simulink model "WebCamTemp"  (Simulink 8.6)
settings: Solver=FixedStepDiscrete  StartTime=0.0  StopTime=Inf  RelTol=1e-3
values from neighbouring files (symbols this model uses):
  gain = 1.0    (= 1)    [WebCamTemp_param.m]
  H = 480    [WebCamTemp_param.m]
  Int = Int/max(max(Int))    [WebCamTemp_param.m]
  maxT = 25    [WebCamTemp_param.m]
  minT = 20    [WebCamTemp_param.m]
  mycmap = [0 0 0 0 0 0 0 0 0 0 0 0 ... (192 elements, 64x3)]    [MyColormaps.mat]
  nAvr = 8    [WebCamTemp_param.m]
  Op = Op/max(max(Op))    [WebCamTemp_param.m]
  T = 0.3    [WebCamTemp_param.m]
  W = 640    [WebCamTemp_param.m]
undefined symbols (not defined in the file or in its folder): IsPositionTracked, IsSkeletonTracked, JointDepthIndices, JointImageIndices, JointTrackingState, JointWorldCoordinates, none, PositionDepthIndices, PositionImageIndices, PositionWorldCoordinates, SegmentationData, serial, SkeletonTrackingID, videoinput
libraries: simulink x20, dspsigops x18, visionsinks x3, instrumentlib x3, visiontextngfix x2, dspstat3 x2, dspmtrx3 x2, visionstatistics x2, dspswit3 x1, powerlib_meascontrol x1, dspvision x1, imaqlib x1
settings Model: Creator=Valentina  LastModifiedBy=VIKTOR
settings OptimizationCC: DefaultParameterBehavior=Inlined
settings DebuggingCC: FcnCallInpInsideContextMsg=UseLocalSettings
settings HardwareCC: ProdBitPerPointer=64  ProdLargestAtomicFloat=Float  ProdIntDivRoundTo=Zero  ProdEndianess=LittleEndian  ProdWordSize=64  ProdHWDeviceType=Intel->x86-64 (Windows64)
settings GRTTargetCC: RTWCAPISignals=on  RTWCAPIParams=on
settings SimEventsCC: propDiagAttribOutput=1  propDiagFcnCallOutput=1  propDiagStatOutput=0  propPreventDuplicateEvents=0

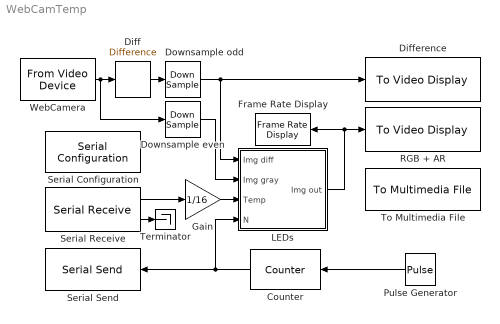
== system WebCamTemp ==
  Counter : dspswit3/Counter  Direction=Up  CountEvent=Rising edge  CounterSize=User defined  MaxCount=5  InitialCount=0  Output=Count  HitValue=32  ResetInput=off  SamplesPerFrame=1  Ts=1/30  CntDtype=uint8  HitDtype=Logical
  Diff : simulink/Discrete/Difference  ICPrevInput=0.0  InputProcessing=Inherited  OutMin=[]  OutMax=[]  OutDataType=fixdt(1, 16)  OutScaling=2^-10  DoSatur=off
  Difference : visionsinks/To Video Display  windowSizeMode=Normal  openAtMdlStart=on  fullScreen=off  videoWindowX=1204  videoWindowY=269  saveWindowSize=off  videoWindowWidth=640  videoWindowHeight=480  inputColorFormat=RGB  inputType=Obsolete  imagePorts=One multidimensional signal  OutputDevice=On-screen video monitor  dataOrg=Column-major  isWindowOpen=off
  "Downsample even " : DownSample
  Downsample odd : DownSample  phase=1
  Frame Rate Display : visionsinks/Frame Rate Display  UpdateRate=10
  Gain : Gain  Gain=1/16  OutDataTypeStr=double
  LEDs : Subsystem
  Pulse Generator : DiscretePulseGenerator  PhaseDelay=2  SampleTime=1/30
  RGB + AR : visionsinks/To Video Display  windowSizeMode=Normal  openAtMdlStart=on  fullScreen=off  videoWindowX=307  videoWindowY=272  saveWindowSize=off  videoWindowWidth=640  videoWindowHeight=480  inputColorFormat=RGB  inputType=Obsolete  imagePorts=One multidimensional signal  OutputDevice=On-screen video monitor  dataOrg=Column-major  isWindowOpen=off
  Serial Configuration : instrumentlib/Serial Configuration  Priority=-200000  ComPortMenu=COM9  ComPort=COM9  ObjConstructor=serial('COM9');  BaudRate=250000  DataBits=8  Parity=none  StopBits=1  FlowControl=none  Timeout=2  ByteOrder=LittleEndian
  Serial Receive : instrumentlib/Serial Receive  ComPortMenu=<Please select a port...>  ComPort=<Please select a port...>  Terminator=<none>  DataSize="[6  1]"  DataType=int16  EnableBlockingMode=off  ActionDataUnavailable=Output last received value  CustomValue=0  SampleTime=1/30
  Serial Send : instrumentlib/Serial Send  ComPortMenu=COM9  ComPort=COM9  ObjConstructor=serial('COM9');  Terminator=<none>  EnableBlockingMode=on
  Terminator : Terminator
  To Multimedia File : dspvision/To Multimedia File  outputFilename=F:\Matlab\WebCamTemp\output.mp4  streamSelection=Video only  videoCompressor=MJPEG Compressor  audioCompressor=None (uncompressed)  imagePorts=One multidimensional signal  fileType=MPEG4  audioDatatype=Determine from input data type  fourcc=RGB  videoQuality=100  mj2000CompFactor=10
  WebCamera : imaqlib/From Video Device  DeviceMenu=winvideo 1 (Webcam C170)  Device=winvideo 1 (Webcam C170)  ObjConstructor=videoinput('winvideo', 1)  VideoFormatMenu=YUY2_640x480  VideoFormat=YUY2_640x480  VideoSource=input1  ROIPosition=[0 0 480 640]  EnableHWTrigger=off  TriggerConfiguration=none/none  SampleTime=1/30  OutputPortsMode=One multidimensional signal  DataType=single  CanDoHWTrigger=no  ReturnedColorSpace=grayscale  BlockHandle=464.0011  ROIWidth=640  ROIHeight=480  ROIColumn=0  ROIRow=0  EngXMLPath=C:\Program Files\MATLAB\R2015b\toolbox\imaq\imaq\private  DevXMLPath=C:\MATLAB\SupportPackages\R2015b\osgenericvideointerface\toolbox\imaq\supportpackages\genericvideo\adaptor\win64  EngLibPath=C:\Program Files\MATLAB\R2015b\toolbox\imaq\imaqblks\imaqmex\win64  ColorSpace=grayscale  BayerSensorAlignment=grbg  AllMetadata=IsPositionTracked;IsSkeletonTracked;JointDepthIndices;JointImageIndices;JointTrackingState;JointWorldCoordinates;PositionDepthIndices;PositionImageIndices;PositionWorldCoordinates;SegmentationData;SkeletonTrackingID
  wires:
  Serial Receive/1 -> Gain/1
  Gain/1 -> LEDs/3(Temp)
  "Downsample even "/1 -> LEDs/2("Img gray ")
  Diff/1 -> Downsample odd/1
  Downsample odd/1 -> Difference/1, LEDs/1(Img diff)
  WebCamera/1 -> Diff/1, "Downsample even "/1
  Pulse Generator/1 -> Counter/1
  LEDs/1(Img out) -> Frame Rate Display/1, RGB + AR/1
  Serial Receive/2 -> Terminator/1
  Counter/1 -> LEDs/4(N), Serial Send/1

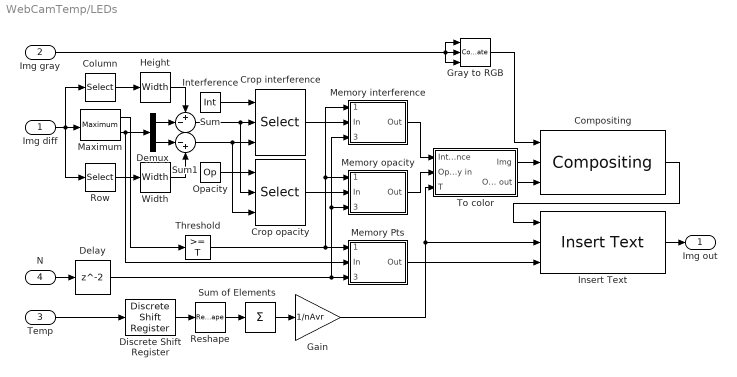
== system WebCamTemp/LEDs ==
  Img diff : Inport
  "Img gray " : Inport  Port=2
  Temp : Inport  Port=3
  N : Inport  Port=4
  Column : Selector  NumberOfDimensions=2  InputPortWidth=3  IndexOptions=Select all,Index vector (dialog)  Indices=1,1  OutputSizes=1,1
  Compositing : visiontextngfix/Compositing  operation=Blend  bFacSrc=Input port  mFacSrc=Specify via dialog  bFactor=0.75  mFactor=1  source=Specify via dialog  coordinates=[1 1]  prodOutputMode=Binary point scaling  prodOutputWordLength=32  prodOutputFracLength=10  roundingMode=Floor  overflowMode=off
  Crop interference : Selector  NumberOfDimensions=2  IndexMode=Zero-based  InputPortWidth=3  IndexOptions=Starting index (port),Starting index (port)  Indices=[1 3],1  OutputSizes=H,W
  Crop opacity : Selector  NumberOfDimensions=2  IndexMode=Zero-based  InputPortWidth=3  IndexOptions=Starting index (port),Starting index (port)  Indices=[1 3],1  OutputSizes=H,W
  Delay : Delay  InitialCondition=0
  Demux : Demux  Outputs=2
  Discrete Shift Register : powerlib_meascontrol/Additional Components/Discrete Shift Register  NSamples=nAvr  InitialValue=0  Ts=-1
  Gain : Gain  Gain=1/nAvr  OutDataTypeStr=single
  Gray to RGB : Concatenate  NumInputs=3  Mode=Multidimensional array  ConcatenateDimension=3
  Height : Width  DataType=uint32
  Insert Text : visiontextngfix/Insert Text  inputType=Obsolete  theText='%4.1f'  getTextLocFrom=Input port  textLoc=[1 1]  getTextColorFrom=Specify via dialog  textColor=[0 0 0]  getTextIntensityFrom=Specify via dialog  textIntensity=0  getTextOpacityFrom=Specify via dialog  textOpacity=1.0  dummyVar2=0  dummyVar3=0  dummyVar4=0  imagePorts=One multidimensional signal  isInputTransposed=off  fontFace=Arial  dummyVar1=0  blockFontSize=24  antiAliased=on
  Interference : Constant  Value=Int  OutDataTypeStr=single
  Maximum : dspstat3/Maximum  fcn=Value and Index  reset=None  indexBase=Zero  operateOver=Entire input  Dimension=1  operation=maximum  roiEnable=off  roiType=Rectangles  roiPortion=Entire ROI  roiOutput=Individual statistics for each ROI  roiFlag=off  accumDataTypeStr=Inherit: Same as product output  accumLastDataTypeStr=Inherit: Same as product output  roundingMode=Floor  overflowMode=off
  Memory interference : Subsystem
  Memory opacity : Subsystem
  Memory Pts : Subsystem
  Opacity : Constant  Value=Op  OutDataTypeStr=single
  Reshape : Reshape  OutputDimensionality=Customize  OutputDimensions=[nAvr,6]
  Row : Selector  NumberOfDimensions=2  InputPortWidth=3  IndexOptions=Index vector (dialog),Select all  Indices=1,1  OutputSizes=1,1
  Sum : Sum  Inputs=+-|
  Sum of Elements : Sum  Inputs=+  CollapseMode=Specified dimension
  Sum1 : Sum  Inputs=|-+
  Threshold : simulink/Logic and Bit Operations/Compare To Constant  relop=>=  const=T  OutDataTypeStr=boolean
  To color : Subsystem
  Width : Width  DataType=uint32
  Img out : Outport
  wires:
  Insert Text/1 -> Img out/1
  Compositing/1 -> Insert Text/1
  To color/2(Opacity out) -> Compositing/3
  Temp/1 -> Discrete Shift Register/1
  To color/1(Img) -> Compositing/2
  Interference/1 -> Crop interference/1
  Demux/2 -> Sum1/1
  Demux/1 -> Sum/2
  Height/1 -> Sum/1
  Sum/1 -> Crop opacity/2, Crop interference/2
  Sum1/1 -> Crop opacity/3, Crop interference/3
  Img diff/1 -> Maximum/1, Column/1, Row/1
  Memory interference/1(Out) -> To color/1(Interference)
  Memory opacity/1(Out) -> To color/2(Opacity in)
  Memory Pts/1(Out) -> Insert Text/3
  Row/1 -> Width/1
  Width/1 -> Sum1/2
  Column/1 -> Height/1
  N/1 -> Delay/1
  Maximum/2 -> Demux/1, Memory Pts/2(In)
  Maximum/1 -> Threshold/1
  Delay/1 -> Memory interference/3(Address), Memory opacity/3(Address), Memory Pts/3(Address)
  Opacity/1 -> Crop opacity/1
  Crop interference/1 -> Memory interference/2(In)
  Crop opacity/1 -> Memory opacity/2(In)
  Sum of Elements/1 -> Gain/1
  Discrete Shift Register/1 -> Reshape/1
  Reshape/1 -> Sum of Elements/1
  Gain/1 -> To color/3(T), Insert Text/2
  "Img gray "/1 -> Gray to RGB/3, Gray to RGB/1, Gray to RGB/2
  Gray to RGB/1 -> Compositing/1
  Threshold/1 -> Memory Pts/1(Enable), Memory interference/1(Enable), Memory opacity/1(Enable)

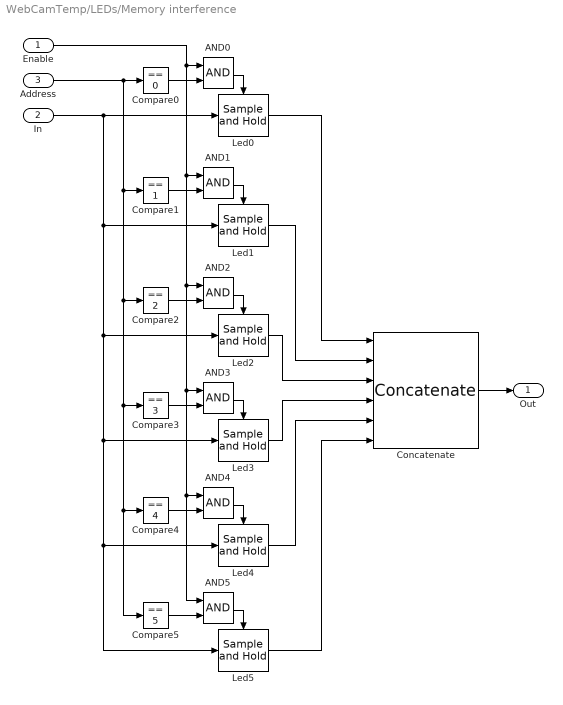
== system WebCamTemp/LEDs/Memory interference ==
  Enable : Inport
  In : Inport  Port=2
  Address : Inport  Port=3
  AND{0..5} (6 alike) : Logic  AllPortsSameDT=off  OutDataTypeStr=boolean
  Compare0 : simulink/Logic and Bit Operations/Compare To Constant  relop===  const=0  OutDataTypeStr=boolean
  Compare1 : simulink/Logic and Bit Operations/Compare To Constant  relop===  const=1  OutDataTypeStr=boolean
  Compare2 : simulink/Logic and Bit Operations/Compare To Constant  relop===  const=2  OutDataTypeStr=boolean
  Compare3 : simulink/Logic and Bit Operations/Compare To Constant  relop===  const=3  OutDataTypeStr=boolean
  Compare4 : simulink/Logic and Bit Operations/Compare To Constant  relop===  const=4  OutDataTypeStr=boolean
  Compare5 : simulink/Logic and Bit Operations/Compare To Constant  relop===  const=5  OutDataTypeStr=boolean
  Concatenate : Concatenate  NumInputs=6  Mode=Multidimensional array  ConcatenateDimension=3
  Led{0..5} (6 alike) : dspsigops/Sample and Hold  trig=Rising edge  initCond=0  latchinput=off
  Out : Outport
  wires:
  Address/1 -> Compare1/1, Compare2/1, Compare3/1, Compare4/1, Compare5/1, Compare0/1
  Concatenate/1 -> Out/1
  In/1 -> Led1/1, Led2/1, Led3/1, Led4/1, Led5/1, Led0/1
  AND0/1 -> Led0/Trigger
  Enable/1 -> AND5/1, AND4/1, AND3/1, AND2/1, AND1/1, AND0/1
  Compare0/1 -> AND0/2
  AND1/1 -> Led1/Trigger
  Compare1/1 -> AND1/2
  AND2/1 -> Led2/Trigger
  Compare2/1 -> AND2/2
  AND3/1 -> Led3/Trigger
  Compare3/1 -> AND3/2
  AND4/1 -> Led4/Trigger
  Compare4/1 -> AND4/2
  AND5/1 -> Led5/Trigger
  Compare5/1 -> AND5/2
  Led5/1 -> Concatenate/6
  Led0/1 -> Concatenate/1
  Led1/1 -> Concatenate/2
  Led4/1 -> Concatenate/5
  Led3/1 -> Concatenate/4
  Led2/1 -> Concatenate/3

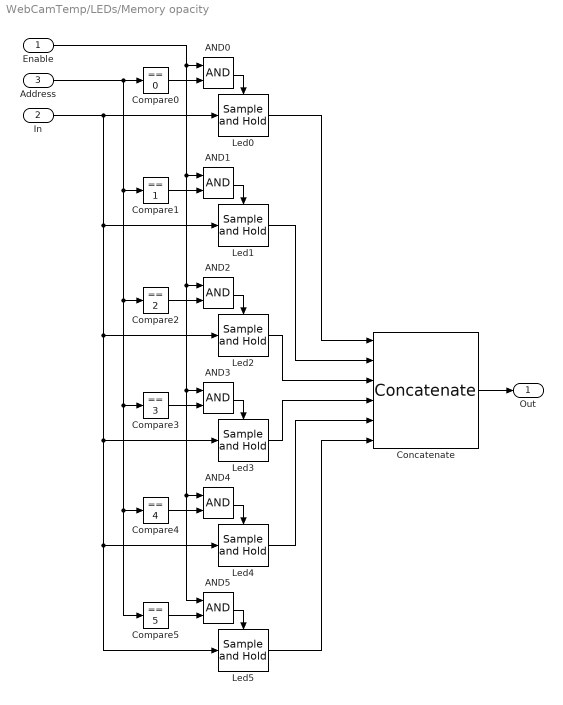
== system WebCamTemp/LEDs/Memory opacity ==
  Enable : Inport
  In : Inport  Port=2
  Address : Inport  Port=3
  AND{0..5} (6 alike) : Logic  AllPortsSameDT=off  OutDataTypeStr=boolean
  Compare0 : simulink/Logic and Bit Operations/Compare To Constant  relop===  const=0  OutDataTypeStr=boolean
  Compare1 : simulink/Logic and Bit Operations/Compare To Constant  relop===  const=1  OutDataTypeStr=boolean
  Compare2 : simulink/Logic and Bit Operations/Compare To Constant  relop===  const=2  OutDataTypeStr=boolean
  Compare3 : simulink/Logic and Bit Operations/Compare To Constant  relop===  const=3  OutDataTypeStr=boolean
  Compare4 : simulink/Logic and Bit Operations/Compare To Constant  relop===  const=4  OutDataTypeStr=boolean
  Compare5 : simulink/Logic and Bit Operations/Compare To Constant  relop===  const=5  OutDataTypeStr=boolean
  Concatenate : Concatenate  NumInputs=6  Mode=Multidimensional array  ConcatenateDimension=3
  Led{0..5} (6 alike) : dspsigops/Sample and Hold  trig=Rising edge  initCond=0  latchinput=off
  Out : Outport
  wires:
  Address/1 -> Compare1/1, Compare2/1, Compare3/1, Compare4/1, Compare5/1, Compare0/1
  Concatenate/1 -> Out/1
  In/1 -> Led1/1, Led2/1, Led3/1, Led4/1, Led5/1, Led0/1
  AND0/1 -> Led0/Trigger
  Enable/1 -> AND5/1, AND4/1, AND3/1, AND2/1, AND1/1, AND0/1
  Compare0/1 -> AND0/2
  AND1/1 -> Led1/Trigger
  Compare1/1 -> AND1/2
  AND2/1 -> Led2/Trigger
  Compare2/1 -> AND2/2
  AND3/1 -> Led3/Trigger
  Compare3/1 -> AND3/2
  AND4/1 -> Led4/Trigger
  Compare4/1 -> AND4/2
  AND5/1 -> Led5/Trigger
  Compare5/1 -> AND5/2
  Led5/1 -> Concatenate/6
  Led0/1 -> Concatenate/1
  Led1/1 -> Concatenate/2
  Led4/1 -> Concatenate/5
  Led3/1 -> Concatenate/4
  Led2/1 -> Concatenate/3

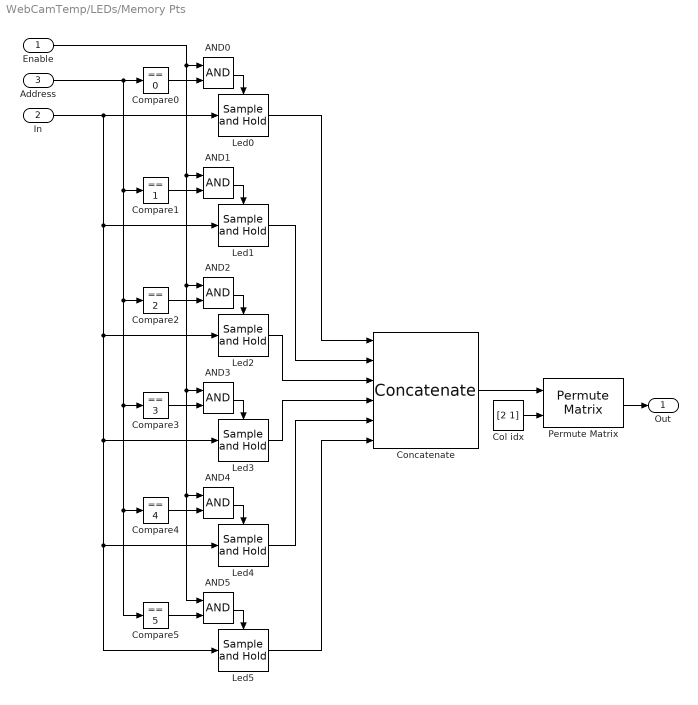
== system WebCamTemp/LEDs/Memory Pts ==
  Enable : Inport
  In : Inport  Port=2
  Address : Inport  Port=3
  AND{0..5} (6 alike) : Logic  AllPortsSameDT=off  OutDataTypeStr=boolean
  Col idx : Constant  Value=[2 1]
  Compare0 : simulink/Logic and Bit Operations/Compare To Constant  relop===  const=0  OutDataTypeStr=boolean
  Compare1 : simulink/Logic and Bit Operations/Compare To Constant  relop===  const=1  OutDataTypeStr=boolean
  Compare2 : simulink/Logic and Bit Operations/Compare To Constant  relop===  const=2  OutDataTypeStr=boolean
  Compare3 : simulink/Logic and Bit Operations/Compare To Constant  relop===  const=3  OutDataTypeStr=boolean
  Compare4 : simulink/Logic and Bit Operations/Compare To Constant  relop===  const=4  OutDataTypeStr=boolean
  Compare5 : simulink/Logic and Bit Operations/Compare To Constant  relop===  const=5  OutDataTypeStr=boolean
  Concatenate : Concatenate  NumInputs=6  Mode=Multidimensional array
  Led{0..5} (6 alike) : dspsigops/Sample and Hold  trig=Rising edge  initCond=0  latchinput=off
  Permute Matrix : dspmtrx3/Permute Matrix  mode=Columns  ZeroOneIdxMode=One-based  errmode=Clip index  checkDims=off
  Out : Outport
  wires:
  Led2/1 -> Concatenate/3
  Led3/1 -> Concatenate/4
  Led4/1 -> Concatenate/5
  Led1/1 -> Concatenate/2
  Led0/1 -> Concatenate/1
  Led5/1 -> Concatenate/6
  Compare5/1 -> AND5/2
  AND5/1 -> Led5/Trigger
  Compare4/1 -> AND4/2
  AND4/1 -> Led4/Trigger
  Compare3/1 -> AND3/2
  AND3/1 -> Led3/Trigger
  Compare2/1 -> AND2/2
  AND2/1 -> Led2/Trigger
  Compare1/1 -> AND1/2
  AND1/1 -> Led1/Trigger
  Compare0/1 -> AND0/2
  Enable/1 -> AND1/1, AND2/1, AND3/1, AND4/1, AND5/1, AND0/1
  AND0/1 -> Led0/Trigger
  In/1 -> Led0/1, Led5/1, Led4/1, Led3/1, Led2/1, Led1/1
  Address/1 -> Compare0/1, Compare5/1, Compare4/1, Compare3/1, Compare2/1, Compare1/1
  Concatenate/1 -> Permute Matrix/1
  Col idx/1 -> Permute Matrix/2
  Permute Matrix/1 -> Out/1

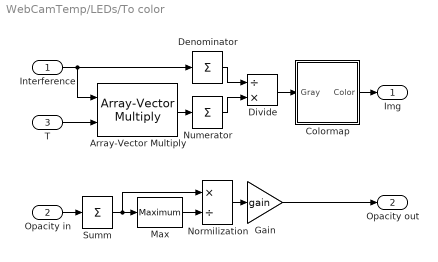
== system WebCamTemp/LEDs/To color ==
  Interference : Inport
  Opacity in : Inport  Port=2
  T : Inport  Port=3
  Array-Vector Multiply : dspmtrx3/Array-Vector Multiply  mode=Mute  saveAsFlag=0  Dimension=3  V_Source=Input port  V_VectFromMask=[0.5 0.25]  firstCoeffSignedness=Auto  firstCoeffDataTypeStr=Inherit: Same word length as input  firstCoeffLastDataTypeStr=Inherit: Same word length as input  firstCoeffMin=[]  firstCoeffMax=[]  outputSignedness=Auto  outputDataTypeStr=Inherit: Same as product output  outputLastDataTypeStr=Inherit: Same as product output  outputMin=[]  outputMax=[]  accumSignedness=Auto  prodOutputSignedness=Auto  roundingMode=Floor  overflowMode=off
  Colormap : Subsystem
  Denominator : Sum  Inputs=+  CollapseMode=Specified dimension  CollapseDim=3  OutDataTypeStr=Inherit: Same as first input
  Divide : Product  Inputs=/*  OutDataTypeStr=Inherit: Same as first input
  Gain : Gain  Gain=gain  OutDataTypeStr=Inherit: Same as input
  Max : dspstat3/Maximum  fcn=Value  reset=None  indexBase=Zero  operateOver=Entire input  Dimension=1  operation=maximum  roiEnable=off  roiType=Rectangles  roiPortion=Entire ROI  roiOutput=Individual statistics for each ROI  roiFlag=off  accumDataTypeStr=Inherit: Same as product output  accumLastDataTypeStr=Inherit: Same as product output  roundingMode=Floor  overflowMode=off
  Normilization : Product  Inputs=*/  OutDataTypeStr=Inherit: Same as first input
  Numerator : Sum  Inputs=+  CollapseMode=Specified dimension  CollapseDim=3  OutDataTypeStr=Inherit: Same as first input
  Summ : Sum  Inputs=+  CollapseMode=Specified dimension  CollapseDim=3  OutDataTypeStr=Inherit: Same as first input
  Img : Outport
  Opacity out : Outport  Port=2
  wires:
  Array-Vector Multiply/1 -> Numerator/1
  Denominator/1 -> Divide/1
  Numerator/1 -> Divide/2
  Divide/1 -> Colormap/1(Gray)
  Interference/1 -> Array-Vector Multiply/1, Denominator/1
  T/1 -> Array-Vector Multiply/2
  Opacity in/1 -> Summ/1
  Summ/1 -> Max/1, Normilization/1
  Gain/1 -> Opacity out/1
  Max/1 -> Normilization/2
  Normilization/1 -> Gain/1
  Colormap/1(Color) -> Img/1

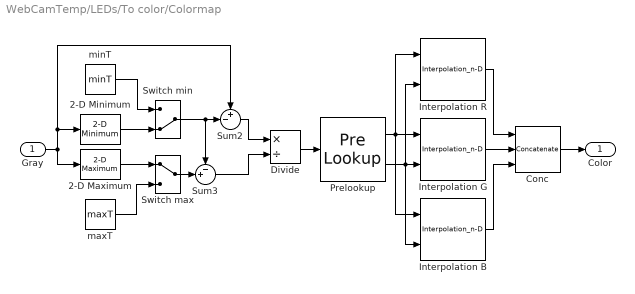
== system WebCamTemp/LEDs/To color/Colormap ==
  Gray : Inport
  2-D Maximum : visionstatistics/2-D Maximum  fcn=Value  reset=None  indexBase=One  operateOver=Entire input  Dimension=1  colComp=on  operation=maximum  roiEnable=off  roiType=Rectangles  roiPortion=Entire ROI  roiOutput=Individual statistics for each ROI  roiFlag=off  accumDataTypeStr=Inherit: Same as product output  accumLastDataTypeStr=Inherit: Same as product output  roundingMode=Floor  overflowMode=off
  2-D Minimum : visionstatistics/2-D Minimum  fcn=Value  reset=None  indexBase=One  operateOver=Entire input  Dimension=1  colComp=on  operation=minimum  roiEnable=off  roiType=Rectangles  roiPortion=Entire ROI  roiOutput=Individual statistics for each ROI  roiFlag=off  accumDataTypeStr=Inherit: Same as product output  accumLastDataTypeStr=Inherit: Same as product output  roundingMode=Floor  overflowMode=off
  Conc : Concatenate  NumInputs=3  Mode=Multidimensional array  ConcatenateDimension=3
  Divide : Product  Inputs=*/  OutDataTypeStr=Inherit: Same as first input
  Interpolation B : Interpolation_n-D  NumberOfTableDimensions=1  Table=mycmap(:,3)  ExtrapMethod=Clip  RemoveProtectionIndex=on  OutDataTypeStr=single  InternalRulePriority=Speed
      settings: InputPortMap=u0,u1
  Interpolation G : Interpolation_n-D  NumberOfTableDimensions=1  Table=mycmap(:,2)  ExtrapMethod=Clip  RemoveProtectionIndex=on  OutDataTypeStr=single  InternalRulePriority=Speed
      settings: InputPortMap=u0,u1
  Interpolation R : Interpolation_n-D  NumberOfTableDimensions=1  Table=mycmap(:,1)  ExtrapMethod=Clip  RemoveProtectionIndex=on  OutDataTypeStr=single  InternalRulePriority=Speed
      settings: InputPortMap=u0,u1
  Prelookup : PreLookup  BreakpointsData=[0:1/63:1]  BeginIndexSearchUsingPreviousIndexResult=on  RemoveProtectionInput=on
  Sum2 : Sum  Inputs=+-|  OutDataTypeStr=Inherit: Same as first input
  Sum3 : Sum  Inputs=-+|  OutDataTypeStr=Inherit: Same as first input
  Switch max : ManualSwitch
  Switch min : ManualSwitch  CurrentSetting=0
  maxT : Constant  Value=maxT  OutDataTypeStr=single
  minT : Constant  Value=minT  OutDataTypeStr=single
  Color : Outport
  wires:
  Sum2/1 -> Divide/1
  Sum3/1 -> Divide/2
  Gray/1 -> 2-D Minimum/1, Sum2/1, 2-D Maximum/1
  Conc/1 -> Color/1
  2-D Minimum/1 -> Switch min/2
  minT/1 -> Switch min/1
  Switch max/1 -> Sum3/2
  2-D Maximum/1 -> Switch max/1
  maxT/1 -> Switch max/2
  Switch min/1 -> Sum2/2, Sum3/1
  Divide/1 -> Prelookup/1
  Prelookup/1 -> Interpolation B/1, Interpolation R/1, Interpolation G/1
  Prelookup/2 -> Interpolation B/2, Interpolation R/2, Interpolation G/2
  Interpolation R/1 -> Conc/1
  Interpolation G/1 -> Conc/2
  Interpolation B/1 -> Conc/3
